simulink model "EPS_sim_test_v1"  (R2019b)
settings: Solver=FixedStepAuto  StartTime=0.0  StopTime=tsimulation  FixedStep=delta_t  MaxStep=10  RelTol=1e-3
values from neighbouring files (symbols this model uses):
  a = 6678    [demoEPS_R2019a.m]    (also in demoEPS_v1.m; demoEPS_v1a.m; demoEPS_v1test.m; demoEPS_v2.m)
  C = Cbat*Nbp*3600    (= 37440)    [demoEPS.m]    (also in demoEPS_R2019a.m; demoEPS_v1.m; demoEPS_v1a.m; demoEPS_v1test.m)
  day = 21    [demoEPS_R2019a.m]    (also in demoEPS_v1.m = 1; demoEPS_v1a.m; demoEPS_v1test.m; demoEPS_v2.m)
  DOD_0 = 0    [demoEPS.m]    (also in demoEPS_R2019a.m; demoEPS_v1.m; demoEPS_v1a.m; demoEPS_v1test.m)
  e = 0.001    [demoEPS_R2019a.m]    (also in demoEPS_v1.m = 0; demoEPS_v1a.m; demoEPS_v1test.m; demoEPS_v2.m)
  hours = 0    [demoEPS_R2019a.m]    (also in demoEPS_v1.m; demoEPS_v1a.m; demoEPS_v1test.m; demoEPS_v2.m)
  i = 51.6    [demoEPS_R2019a.m]    (also in demoEPS_v1.m; demoEPS_v1a.m; demoEPS_v1test.m; demoEPS_v2.m)
  I_BC_max = -input (4)    [battchargedischarge.m]    (also in demoEPS.m = 3; demoEPS_R2019a.m = 3; demoEPS_v1.m = 3; demoEPS_v1a.m = 3)
  I_BD_max = input (3)    [battchargedischarge.m]    (also in demoEPS.m = 5; demoEPS_R2019a.m = 5; demoEPS_v1.m = 5; demoEPS_v1a.m = 5)
  m = 10    [demoEPS_R2019a.m]    (also in demoEPS_v1.m; demoEPS_v1a.m; demoEPS_v1test.m; demoEPS_v2.m)
  minutes = 0    [demoEPS_R2019a.m]    (also in demoEPS_v1.m; demoEPS_v1a.m; demoEPS_v1test.m; demoEPS_v2.m)
  month = 3    [demoEPS_R2019a.m]    (also in demoEPS_v1.m = 1; demoEPS_v1a.m = 6; demoEPS_v1test.m = 12; demoEPS_v2.m)
  Nbs = math.ceil(Vbusmin/Vbatmin)    [calc_mass_EPS.m]    (also in demoEPS.m = 4; demoEPS_R2019a.m = 4; demoEPS_v1.m = 4; demoEPS_v1a.m = 4)
  nu = 0    [demoEPS_R2019a.m]    (also in demoEPS_v1.m; demoEPS_v1a.m; demoEPS_v1test.m; demoEPS_v2.m)
  O = 300    [demoEPS_R2019a.m]    (also in demoEPS_v1.m = 185; demoEPS_v1a.m = 69; demoEPS_v1test.m = 180; demoEPS_v2.m = 243)
  o = 90    [demoEPS_R2019a.m]    (also in demoEPS_v1.m; demoEPS_v1a.m = 150; demoEPS_v1test.m = 150; demoEPS_v2.m)
  P_eps = 0.6    [demoEPS.m]    (also in demoEPS_R2019a.m; demoEPS_v1.m; demoEPS_v1a.m; demoEPS_v1test.m)
  Pload1 = 50    [demoEPS.m]    (also in demoEPS_R2019a.m; demoEPS_v1.m; demoEPS_v1a.m; demoEPS_v1test.m)
  Pload2 = 2    [demoEPS.m]    (also in demoEPS_R2019a.m; demoEPS_v1.m; demoEPS_v1a.m; demoEPS_v1test.m)
  Pload3 = 2.5    [demoEPS.m]    (also in demoEPS_R2019a.m; demoEPS_v1.m; demoEPS_v1a.m; demoEPS_v1test.m)
  Pload4 = 1.7    [demoEPS.m]    (also in demoEPS_R2019a.m; demoEPS_v1.m; demoEPS_v1a.m; demoEPS_v1test.m)
  Psa = 48    [demoEPS.m]    (also in demoEPS_R2019a.m; demoEPS_v1.m; demoEPS_v1a.m; demoEPS_v1test.m)
  seconds = 0    [demoEPS_R2019a.m]    (also in demoEPS_v1.m; demoEPS_v1a.m; demoEPS_v1test.m; demoEPS_v2.m)
  Torbit = 2*pi*sqrt(((h+6378)^3)/398600)/60    [calc_mass_EPS.m]    (also in demoEPS.m = 5400; demoEPS_R2019a.m = 2*pi*sqrt(a^3/(3.986004418E5)); demoEPS_v1.m = 5400; demoEPS_v1a.m = 2*pi*sqrt(a^3/(3.986004418E5)))
  year = 2020    [demoEPS_R2019a.m]    (also in demoEPS_v1.m; demoEPS_v1a.m = 2019; demoEPS_v1test.m = 2019; demoEPS_v2.m)
undefined symbols (not defined in the file or in its folder): km, s
libraries: aerolibconvert2 x6, dspmathops x4, vrlib x3, simulink x2, aerolibutil x2, sharedtransform x1, aerolibgravity2 x1, aerolibcelestial x1
settings Model: Creator=Ricardo  LastModifiedBy=Ricardo

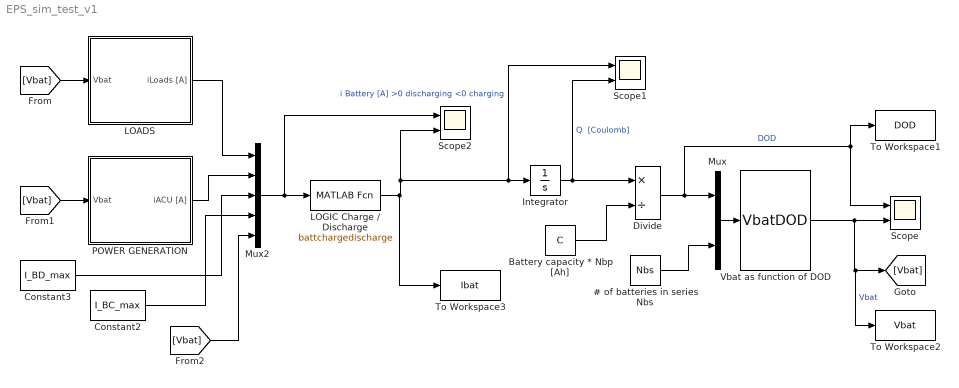
== system EPS_sim_test_v1 ==
  # of batteries in series Nbs : Constant  Value=Nbs
  Battery capacity * Nbp [Ah] : Constant  Value=C
  Constant2 : Constant  Value=I_BC_max
  Constant3 : Constant  Value=I_BD_max
  Divide : Product  Inputs=*/
  Integrator : Integrator  InitialCondition=DOD_0
  LOADS : Subsystem
  LOGIC Charge / Discharge : MATLABFcn  MATLABFcn=battchargedischarge
  Mux : Mux  Inputs=2
  Mux2 : Mux  Inputs=5
  POWER GENERATION : Subsystem
  Scope : Scope  NumInputPorts=2
  Scope1 : Scope  NumInputPorts=2
  Scope2 : Scope  NumInputPorts=2
  To Workspace1 : ToWorkspace  VariableName=DOD  SaveFormat=Timeseries  SampleTime=-1
  To Workspace2 : ToWorkspace  VariableName=Vbat  SaveFormat=Timeseries  SampleTime=-1
  To Workspace3 : ToWorkspace  VariableName=Ibat  SaveFormat=Timeseries  SampleTime=-1
  Vbat as function of DOD : MATLABFcn  MATLABFcn=VbatDOD
  wires:
  Mux/1 -> Vbat as function of DOD/1
  # of batteries in series Nbs/1 -> Mux/2
  Vbat as function of DOD/1 -> To Workspace2/1, [Vbat], Scope/2  "Vbat"
  Divide/1 -> To Workspace1/1, Scope/1, Mux/1  "DOD"
  Integrator/1 -> Scope1/2, Divide/1  "Q  [Coulomb]"
  Battery capacity * Nbp [Ah]/1 -> Divide/2
  [Vbat] -> LOADS/1(Vbat)
  POWER GENERATION/1(iACU [A]) -> Mux2/2
  [Vbat] -> POWER GENERATION/1(Vbat)
  LOADS/1(iLoads [A]) -> Mux2/1
  Mux2/1 -> LOGIC Charge / Discharge/1, Scope2/1
  Constant3/1 -> Mux2/3
  Constant2/1 -> Mux2/4
  LOGIC Charge / Discharge/1 -> To Workspace3/1, Scope1/1, Integrator/1, Scope2/2  "i Battery [A] >0 discharging <0 charging"
  [Vbat] -> Mux2/5

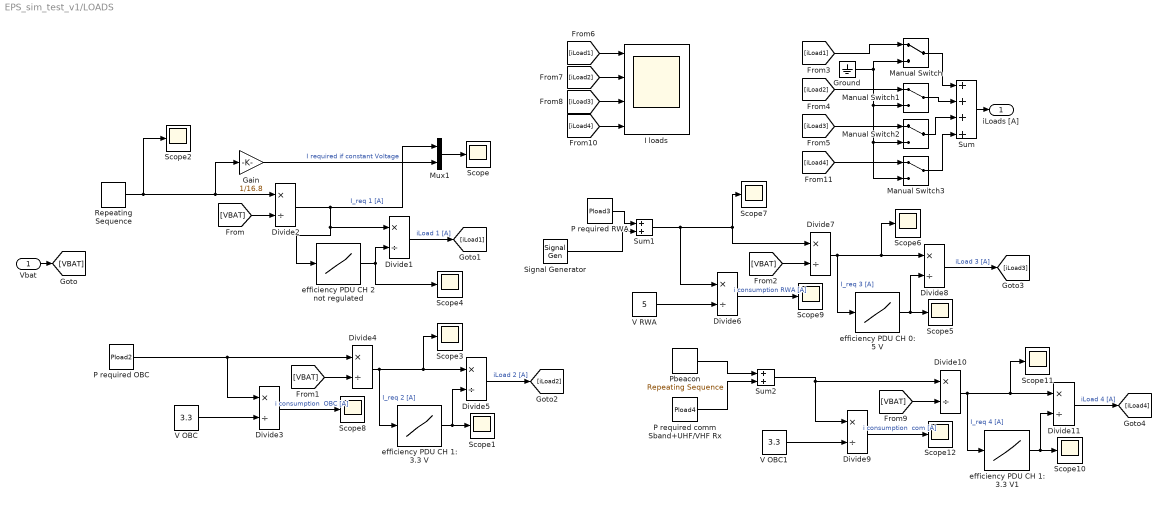
== system EPS_sim_test_v1/LOADS ==
  Vbat : Inport
  Divide{1..11} (11 alike) : Product  Inputs=*/
  Gain : Gain  Gain=1/16.8
  Ground : Ground
  I loads : Scope  NumInputPorts=4
  Manual Switch{,1..3} (4 alike) : ManualSwitch
  Mux1 : Mux  Inputs=2
  P required OBC : Constant  Value=Pload2
  P required RWA : Constant  Value=Pload3
  P required comm Sband+UHF/VHF Rx : Constant  Value=Pload4
  Pbeacon : simulink/Sources/Repeating Sequence  rep_seq_t=[0, 1, 21, 22, 200]  rep_seq_y=[0 3.3 3.3 0 0]
  Repeating Sequence : simulink/Sources/Repeating Sequence  rep_seq_t=[0, 1, (Torbit/2),(Torbit/2)+1, Torbit,2*Torbit,3*Torbit,4*Torbit]  rep_seq_y=[0.32 Pload1 Pload1 0.32 0.32 0.32 0.32 0.32]
  Scope{,1..12} (13 alike) : Scope
  Signal Generator : SignalGenerator  WaveForm=random  Amplitude=0.6  Frequency=0.01
  Sum : Sum  Inputs=++++
  Sum1 : Sum
  Sum2 : Sum
  V OBC : Constant  Value=3.3
  V OBC1 : Constant  Value=3.3
  V RWA : Constant  Value=5
  efficiency PDU CH 0: 5 V : Lookup_n-D  NumberOfTableDimensions=1  BreakpointsForDimension1=[0,0.15,0.18,0.25,0.4,0.5,0.75,1,1.5,2]  Table=[0,0.65,0.7,0.8,0.85,0.88,0.89,0.9,0.88,0.87]  InternalRulePriority=Speed  RndMeth=Simplest  InputSameDT=on
  efficiency PDU CH 1: 3.3 V : Lookup_n-D  NumberOfTableDimensions=1  BreakpointsForDimension1=[0,0.15,0.18,0.25,0.4,0.5,0.75,1,1.5,2]  Table=[0,0.65,0.7,0.8,0.85,0.88,0.89,0.9,0.88,0.87]  InternalRulePriority=Speed  RndMeth=Simplest  InputSameDT=on
  efficiency PDU CH 1: 3.3 V1 : Lookup_n-D  NumberOfTableDimensions=1  BreakpointsForDimension1=[0,0.15,0.18,0.25,0.4,0.5,0.75,1,1.5,2]  Table=[0,0.65,0.7,0.8,0.85,0.88,0.89,0.9,0.88,0.87]  InternalRulePriority=Speed  RndMeth=Simplest  InputSameDT=on
  efficiency PDU CH 2 not regulated : Lookup_n-D  NumberOfTableDimensions=1  BreakpointsForDimension1=[0,0.15,0.2,0.25,0.4,0.5,0.75,1,1.5,2]  Table=[0.25,0.97,0.99,0.98594,0.97572,0.96294,0.95783,0.95783,0.94505,0.93994]  InternalRulePriority=Speed  RndMeth=Simplest  InputSameDT=on
  iLoads [A] : Outport
  wires:
  Gain/1 -> Mux1/2  "I required if constant Voltage"
  Divide2/1 -> Mux1/1, efficiency PDU CH 2 not regulated/1, Divide1/1  "I_req 1 [A]"
  P required OBC/1 -> Divide4/1, Divide3/1
  V OBC/1 -> Divide3/2
  Vbat/1 -> [VBAT]
  [VBAT] -> Divide2/2
  [VBAT] -> Divide4/2
  Divide4/1 -> efficiency PDU CH 1: 3.3 V/1, Scope3/1, Divide5/1  "I_req 2 [A]"
  Sum/1 -> iLoads [A]/1
  Mux1/1 -> Scope/1
  efficiency PDU CH 1: 3.3 V/1 -> Scope1/1, Divide5/2
  Repeating Sequence/1 -> Scope2/1, Gain/1, Divide2/1
  efficiency PDU CH 2 not regulated/1 -> Scope4/1, Divide1/2
  Divide1/1 -> [iLoad1]  "iLoad 1 [A]"
  Divide5/1 -> [iLoad2]  "iLoad 2 [A]"
  V RWA/1 -> Divide6/2
  Divide7/1 -> efficiency PDU CH 0: 5 V/1, Scope6/1, Divide8/1  "I_req 3 [A]"
  efficiency PDU CH 0: 5 V/1 -> Scope5/1, Divide8/2
  [VBAT] -> Divide7/2
  Divide8/1 -> [iLoad3]  "iLoad 3 [A]"
  Manual Switch/1 -> Sum/1
  Manual Switch1/1 -> Sum/2
  Manual Switch2/1 -> Sum/3
  [iLoad2] -> I loads/2
  [iLoad1] -> I loads/1
  [iLoad3] -> I loads/3
  Sum1/1 -> Divide6/1, Divide7/1, Scope7/1
  P required RWA/1 -> Sum1/1
  Signal Generator/1 -> Sum1/2
  Divide3/1 -> Scope8/1  "i consumption  OBC [A]"
  Divide6/1 -> Scope9/1  "i consumption RWA [A]"
  Divide9/1 -> Scope12/1  "i consumption  com [A]"
  [VBAT] -> Divide10/2
  Divide11/1 -> [iLoad4]  "iLoad 4 [A]"
  efficiency PDU CH 1: 3.3 V1/1 -> Scope10/1, Divide11/2
  Divide10/1 -> efficiency PDU CH 1: 3.3 V1/1, Scope11/1, Divide11/1  "I_req 4 [A]"
  Sum2/1 -> Divide9/1, Divide10/1
  V OBC1/1 -> Divide9/2
  [iLoad4] -> I loads/4
  Manual Switch3/1 -> Sum/4
  P required comm Sband+UHF/VHF Rx/1 -> Sum2/2
  Pbeacon/1 -> Sum2/1
  [iLoad4] -> Manual Switch3/1
  [iLoad3] -> Manual Switch2/1
  [iLoad2] -> Manual Switch1/1
  [iLoad1] -> Manual Switch/1
  Ground/1 -> Manual Switch/2, Manual Switch3/2, Manual Switch2/2, Manual Switch1/2

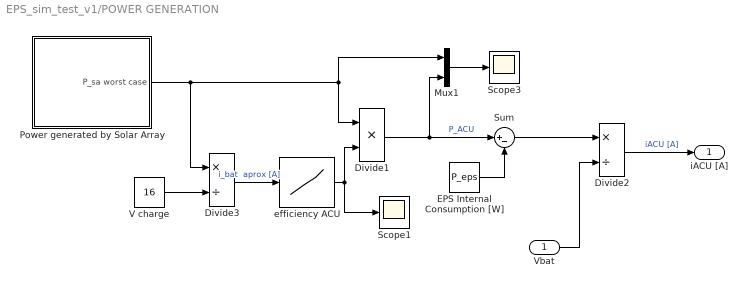
== system EPS_sim_test_v1/POWER GENERATION ==
  Vbat : Inport
  Divide1 : Product  Inputs=**
  Divide2 : Product  Inputs=*/
  Divide3 : Product  Inputs=*/
  EPS Internal Consumption [W] : Constant  Value=P_eps
  Mux1 : Mux  Inputs=2
  Power generated by Solar Array : Subsystem
  Scope1 : Scope
  Scope3 : Scope
  Sum : Sum  Inputs=|+-
  V charge : Constant  Value=16
  efficiency ACU : Lookup_n-D  NumberOfTableDimensions=1  BreakpointsForDimension1=[0,0.15,0.18,0.25,0.4,0.5,0.75,1,1.5,2]  Table=[0,0.59377,0.7,0.75479,0.79162,0.8238,0.85831,0.86406,0.85256,0.84681]  InternalRulePriority=Speed  RndMeth=Simplest  InputSameDT=on
  iACU [A] : Outport
  wires:
  Divide2/1 -> iACU [A]/1  "iACU [A]"
  Mux1/1 -> Scope3/1
  Vbat/1 -> Divide2/2
  efficiency ACU/1 -> Scope1/1, Divide1/2
  Divide1/1 -> Sum/1, Mux1/2  "P_ACU"
  Sum/1 -> Divide2/1
  EPS Internal Consumption [W]/1 -> Sum/2
  Divide3/1 -> efficiency ACU/1  "i_bat  aprox [A]"
  V charge/1 -> Divide3/2
  Power generated by Solar Array/1(P_sa worst case) -> Divide3/1, Mux1/1, Divide1/1

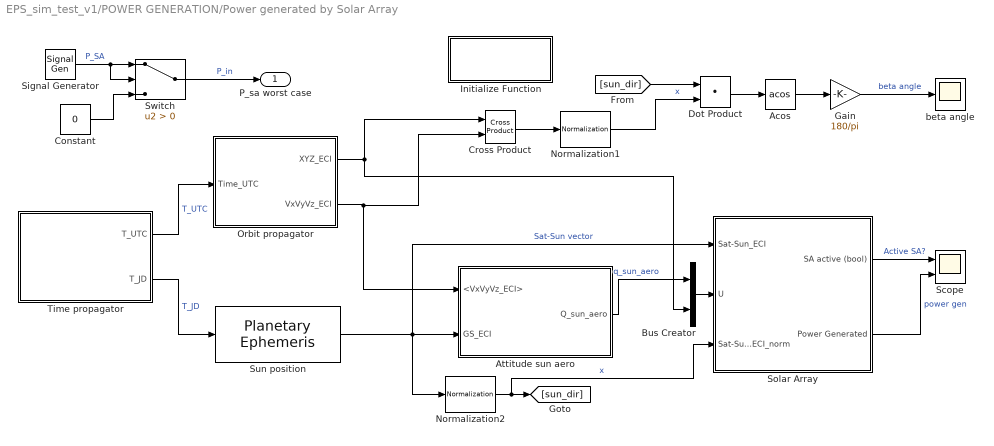
== system EPS_sim_test_v1/POWER GENERATION/Power generated by Solar Array ==
  Acos : Trigonometry  Operator=acos
  Attitude sun aero : Subsystem
  Bus Creator : BusCreator  Inputs=2
  Constant : Constant  Value=0
  Cross Product : vrlib/Utilities/Cross Product
      settings: SourceProductName=Simulink
  Dot Product : DotProduct  InputSameDT=on  OutDataTypeStr=Inherit: Inherit via internal rule
  Gain : Gain  Gain=180/pi
  Initialize Function : Subsystem  TreatAsAtomicUnit=on
  Normalization1 : dspmathops/Normalization  NormType=2-norm  Bias=1e-10  NormOver=Each column  Dimension=1  roundingMode=Floor  overflowMode=off  accumDataTypeStr=Inherit: Same as product output  accumLastDataTypeStr=Inherit: Same as product output  outputDataTypeStr=Inherit: Same as product output  outputMin=[]  outputMax=[]  outputLastDataTypeStr=Inherit: Same as product output
      settings: SourceProductName=DSP System Toolbox
  Normalization2 : dspmathops/Normalization  NormType=2-norm  Bias=1e-10  NormOver=Each column  Dimension=1  roundingMode=Floor  overflowMode=off  accumDataTypeStr=Inherit: Same as product output  accumLastDataTypeStr=Inherit: Same as product output  outputDataTypeStr=Inherit: Same as product output  outputMin=[]  outputMax=[]  outputLastDataTypeStr=Inherit: Same as product output
      settings: SourceProductName=DSP System Toolbox
  Orbit propagator : Subsystem
  Scope : Scope  NumInputPorts=2
  Signal Generator : SignalGenerator  Amplitude=-Psa  Frequency=1/Torbit
  Solar Array : Subsystem
  Sun position : aerolibcelestial/Planetary Ephemeris  kmflag=km,km/s  epochflag=Julian date  de=DE405  nCenter=Earth  nTarget=Sun  errorflag=Error  velflag=off
      settings: SourceProductName=Aerospace Blockset  SourceProductBaseCode=AE
  Switch : Switch  Criteria=u2 > Threshold
  Time propagator : Subsystem
  beta angle : Scope
  P_sa worst case : Outport
  wires:
  Signal Generator/1 -> Switch/2, Switch/1  "P_SA"
  Constant/1 -> Switch/3
  Gain/1 -> beta angle/1  "beta angle"
  Cross Product/1 -> Normalization1/1
  Acos/1 -> Gain/1
  Dot Product/1 -> Acos/1
  Bus Creator/1 -> Solar Array/2(U)
  Orbit propagator/1(XYZ_ECI) -> Cross Product/1, Bus Creator/2
  [sun_dir] -> Dot Product/1
  Time propagator/2(T_JD) -> Sun position/1  "T_JD"
  Normalization2/1 -> Solar Array/3(Sat-Sun_ECI_norm), [sun_dir]  "x"
  Attitude sun aero/1(Q_sun_aero) -> Bus Creator/1  "q_sun_aero"
  Normalization1/1 -> Dot Product/2  "x"
  Time propagator/1(T_UTC) -> Orbit propagator/1("Time_UTC ")  "T_UTC"
  Sun position/1 -> Normalization2/1, Solar Array/1(Sat-Sun_ECI), Attitude sun aero/2(GS_ECI)  "Sat-Sun vector"
  Solar Array/1(SA active (bool)) -> Scope/1  "Active SA?"
  Orbit propagator/2(VxVyVz_ECI) -> Cross Product/2, Attitude sun aero/1(<VxVyVz_ECI>)
  Solar Array/2(Power Generated) -> Scope/2  "power gen"
  Switch/1 -> P_sa worst case/1  "P_in"

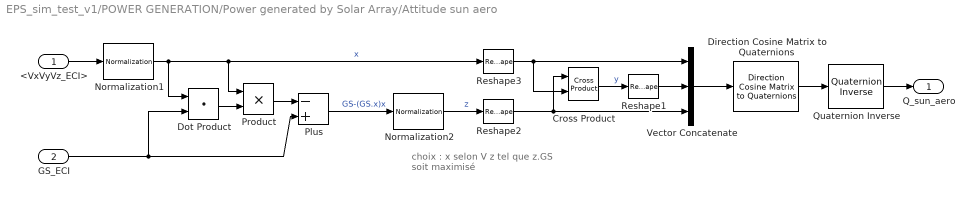
== system EPS_sim_test_v1/POWER GENERATION/Power generated by Solar Array/Attitude sun aero ==
  note: choix :
      | x selon V
      | z tel que z.GS soit maximisé
  <VxVyVz_ECI> : Inport
  GS_ECI : Inport  Port=2
  Cross Product : vrlib/Utilities/Cross Product
      settings: SourceProductName=Simulink
  Direction Cosine Matrix to Quaternions : sharedtransform/Direction Cosine Matrix  to Quaternions  aMode=0  action=None  tolerance=eps(2)
      settings: SourceProductName=Aerospace Blockset  SourceProductBaseCode=AE
  Dot Product : DotProduct  InputSameDT=on  OutDataTypeStr=Inherit: Inherit via internal rule
  Normalization1 : dspmathops/Normalization  NormType=2-norm  Bias=1e-10  NormOver=Each column  Dimension=1  roundingMode=Floor  overflowMode=off  accumDataTypeStr=Inherit: Same as product output  accumLastDataTypeStr=Inherit: Same as product output  outputDataTypeStr=Inherit: Same as product output  outputMin=[]  outputMax=[]  outputLastDataTypeStr=Inherit: Same as product output
      settings: SourceProductName=DSP System Toolbox
  Normalization2 : dspmathops/Normalization  NormType=2-norm  Bias=1e-10  NormOver=Each column  Dimension=1  roundingMode=Floor  overflowMode=off  accumDataTypeStr=Inherit: Same as product output  accumLastDataTypeStr=Inherit: Same as product output  outputDataTypeStr=Inherit: Same as product output  outputMin=[]  outputMax=[]  outputLastDataTypeStr=Inherit: Same as product output
      settings: SourceProductName=DSP System Toolbox
  Plus : Sum  Inputs=-+
  Product : Product
  Quaternion Inverse : aerolibutil/Quaternion Inverse
      settings: SourceProductName=Aerospace Blockset
  Reshape1 : Reshape  OutputDimensionality=Column vector (2-D)
  Reshape2 : Reshape  OutputDimensionality=Column vector (2-D)
  Reshape3 : Reshape  OutputDimensionality=Column vector (2-D)
  Vector Concatenate : Concatenate  NumInputs=3  Mode=Multidimensional array  ConcatenateDimension=2
  Q_sun_aero : Outport  VectorParamsAs1DForOutWhenUnconnected=off
  wires:
  Quaternion Inverse/1 -> Q_sun_aero/1
  Reshape2/1 -> Vector Concatenate/3, Cross Product/1
  Reshape3/1 -> Vector Concatenate/1, Cross Product/2
  Product/1 -> Plus/1
  Dot Product/1 -> Product/2
  Cross Product/1 -> Reshape1/1  "y"
  Normalization2/1 -> Reshape2/1  "z"
  Plus/1 -> Normalization2/1  "GS-(GS.x)x"
  GS_ECI/1 -> Dot Product/2, Plus/2
  Vector Concatenate/1 -> Direction Cosine Matrix to Quaternions/1
  Direction Cosine Matrix to Quaternions/1 -> Quaternion Inverse/1
  Normalization1/1 -> Dot Product/1, Product/1, Reshape3/1  "x"
  <VxVyVz_ECI>/1 -> Normalization1/1
  Reshape1/1 -> Vector Concatenate/2

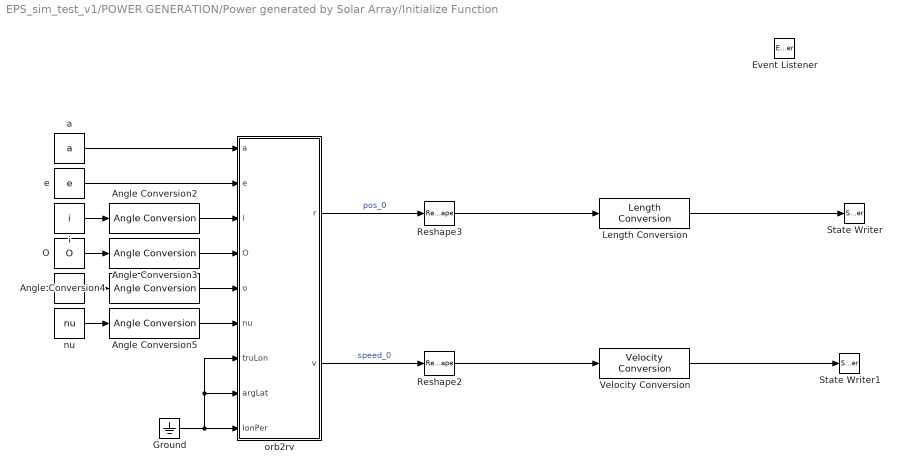
== system EPS_sim_test_v1/POWER GENERATION/Power generated by Solar Array/Initialize Function ==
  Angle Conversion{2..5} (4 alike) : aerolibconvert2/Angle Conversion  IU=deg  OU=rad
  Event Listener : EventListener  DisableCoverage=on  EventName=reset
  Ground : Ground
  Length Conversion : aerolibconvert2/Length Conversion  IU=km  OU=m
  O : Constant  Value=O
  Reshape2 : Reshape  OutputDimensionality=Column vector (2-D)
  Reshape3 : Reshape  OutputDimensionality=Column vector (2-D)
  State Writer : StateWriter  StateOwnerBlock=../../Orbit propagator/Integrator_pos
  State Writer1 : StateWriter  StateOwnerBlock=../../Orbit propagator/Integrator_speed
  Velocity Conversion : aerolibconvert2/Velocity Conversion  IU=km/s  OU=m/s
  a : Constant  Value=a
  e : Constant  Value=e
  i : Constant  Value=i
  nu : Constant  Value=nu
  o : Constant  Value=o
  orb2rv : MATLAB Function  TreatAsAtomicUnit=on
  wires:
  Angle Conversion2/1 -> orb2rv/3(i)
  Length Conversion/1 -> State Writer/1
  Angle Conversion4/1 -> orb2rv/5(o)
  nu/1 -> Angle Conversion5/1
  Angle Conversion3/1 -> orb2rv/4(O)
  e/1 -> orb2rv/2(e)
  Reshape3/1 -> Length Conversion/1
  O/1 -> Angle Conversion3/1
  a/1 -> orb2rv/1(a)
  i/1 -> Angle Conversion2/1
  orb2rv/1(r) -> Reshape3/1  "pos_0"
  o/1 -> Angle Conversion4/1
  Angle Conversion5/1 -> orb2rv/6(nu)
  Velocity Conversion/1 -> State Writer1/1
  Reshape2/1 -> Velocity Conversion/1
  orb2rv/2(v) -> Reshape2/1  "speed_0"
  Ground/1 -> orb2rv/8(argLat), orb2rv/7(truLon), orb2rv/9(lonPer)

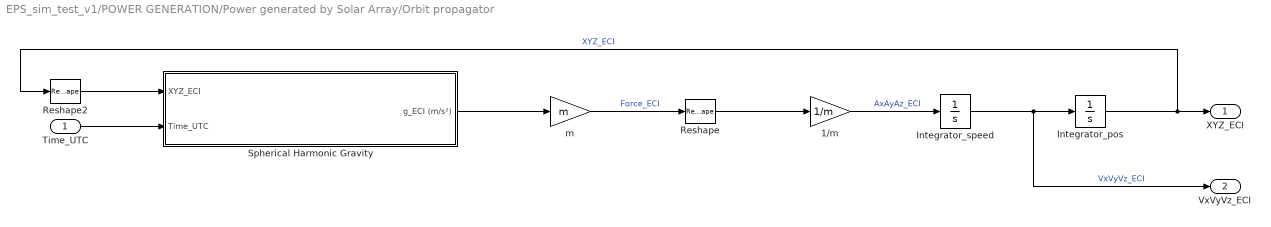
== system EPS_sim_test_v1/POWER GENERATION/Power generated by Solar Array/Orbit propagator ==
  "Time_UTC " : Inport
  1/m : Gain  Gain=1/m
  Integrator_pos : Integrator
  Integrator_speed : Integrator
  Reshape : Reshape  OutputDimensionality=Column vector (2-D)
  Reshape2 : Reshape  OutputDimensionality=Column vector (2-D)
  Spherical Harmonic Gravity : Subsystem  TreatAsAtomicUnit=on  SystemSampleTime=1
  m : Gain  Gain=m
  XYZ_ECI : Outport  VectorParamsAs1DForOutWhenUnconnected=off
  VxVyVz_ECI : Outport  Port=2
  wires:
  Integrator_pos/1 -> Reshape2/1, XYZ_ECI/1  "XYZ_ECI"
  Integrator_speed/1 -> VxVyVz_ECI/1, Integrator_pos/1  "VxVyVz_ECI"
  1/m/1 -> Integrator_speed/1  "AxAyAz_ECI"
  Reshape/1 -> 1/m/1
  m/1 -> Reshape/1  "Force_ECI"
  Spherical Harmonic Gravity/1(g_ECI (m/s²)) -> m/1
  "Time_UTC "/1 -> Spherical Harmonic Gravity/2(Time_UTC)
  Reshape2/1 -> Spherical Harmonic Gravity/1(XYZ_ECI)

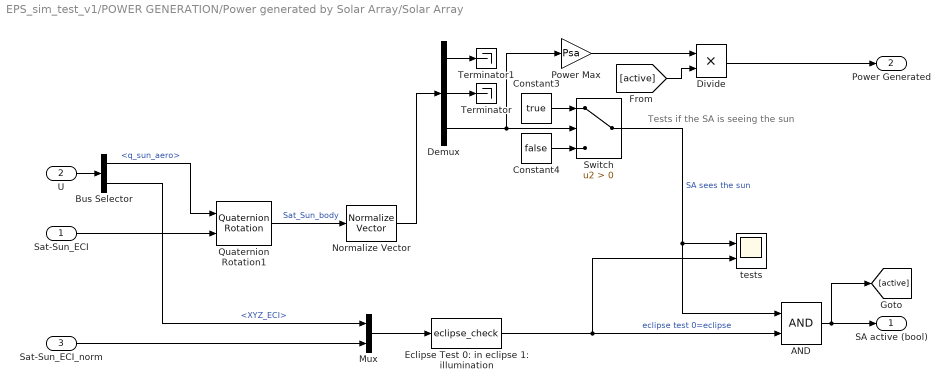
== system EPS_sim_test_v1/POWER GENERATION/Power generated by Solar Array/Solar Array ==
  note: Tests if the SA is seeing the sun
  Sat-Sun_ECI : Inport
  U : Inport  Port=2
  Sat-Sun_ECI_norm : Inport  Port=3
  AND : Logic  IconShape=distinctive  AllPortsSameDT=off  OutDataTypeStr=boolean
  Bus Selector : BusSelector  OutputSignals=q_sun_aero,XYZ_ECI
  Constant3 : Constant  Value=true
  Constant4 : Constant  Value=false
  Demux : Demux  Outputs=3
  Divide : Product  Inputs=**
  Eclipse Test 0: in eclipse 1: illumination : MATLABFcn  MATLABFcn=eclipse_check
  Mux : Mux  Inputs=2
  Normalize Vector : vrlib/Utilities/Normalize Vector  maxzero=0
      settings: SourceProductName=Simulink
  Power Max : Gain  Gain=Psa
  Quaternion Rotation1 : aerolibutil/Quaternion Rotation
  Switch : Switch  Criteria=u2 > Threshold
  Terminator : Terminator
  Terminator1 : Terminator
  tests : Scope  NumInputPorts=2
  SA active (bool) : Outport  VectorParamsAs1DForOutWhenUnconnected=off
  Power Generated : Outport  Port=2
  wires:
  Switch/1 -> AND/1, tests/1  "SA sees the sun"
  U/1 -> Bus Selector/1
  Sat-Sun_ECI/1 -> Quaternion Rotation1/2
  Bus Selector/1 -> Quaternion Rotation1/1  "<q_sun_aero>"
  Quaternion Rotation1/1 -> Normalize Vector/1  "Sat_Sun_body"
  Demux/3 -> Power Max/1, Switch/2
  Constant3/1 -> Switch/1
  Demux/2 -> Terminator/1
  Demux/1 -> Terminator1/1
  Bus Selector/2 -> Mux/1  "<XYZ_ECI>"
  AND/1 -> SA active (bool)/1, [active]
  Constant4/1 -> Switch/3
  Normalize Vector/1 -> Demux/1
  Divide/1 -> Power Generated/1
  Power Max/1 -> Divide/1
  [active] -> Divide/2
  Sat-Sun_ECI_norm/1 -> Mux/2
  Mux/1 -> Eclipse Test 0: in eclipse 1: illumination/1
  Eclipse Test 0: in eclipse 1: illumination/1 -> AND/2, tests/2  "eclipse test 0=eclipse"

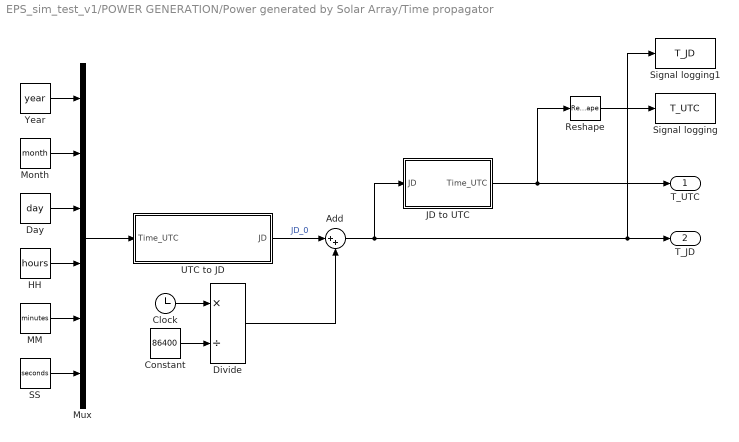
== system EPS_sim_test_v1/POWER GENERATION/Power generated by Solar Array/Time propagator ==
  Add : Sum  Inputs=|++
  Clock : Clock
  Constant : Constant  Value=86400
  Day : Constant  Value=day
  Divide : Product  Inputs=*/
  HH : Constant  Value=hours
  JD to UTC : MATLAB Function  TreatAsAtomicUnit=on
  MM : Constant  Value=minutes
  Month : Constant  Value=month
  Mux : Mux  Inputs=6
  Reshape : Reshape
  SS : Constant  Value=seconds
  Signal logging : ToWorkspace  VariableName=T_UTC  SaveFormat=Timeseries  SampleTime=1
      settings: Save2DSignal=2-D array (concatenate along first dimension)
  Signal logging1 : ToWorkspace  VariableName=T_JD  SaveFormat=Timeseries  SampleTime=1
      settings: Save2DSignal=2-D array (concatenate along first dimension)
  UTC to JD : MATLAB Function  TreatAsAtomicUnit=on
  Year : Constant  Value=year
  T_UTC : Outport  VectorParamsAs1DForOutWhenUnconnected=off
  T_JD : Outport  Port=2  VectorParamsAs1DForOutWhenUnconnected=off
  wires:
  UTC to JD/1(JD) -> Add/1  "JD_0"
  Clock/1 -> Divide/1
  Constant/1 -> Divide/2
  JD to UTC/1(Time_UTC) -> T_UTC/1, Reshape/1
  Divide/1 -> Add/2
  Mux/1 -> UTC to JD/1(Time_UTC)
  Day/1 -> Mux/3
  Month/1 -> Mux/2
  Year/1 -> Mux/1
  HH/1 -> Mux/4
  MM/1 -> Mux/5
  SS/1 -> Mux/6
  Reshape/1 -> Signal logging/1
  Add/1 -> Signal logging1/1, T_JD/1, JD to UTC/1(JD)

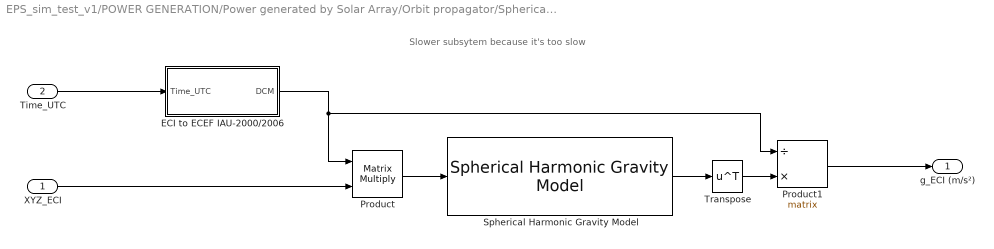
== system EPS_sim_test_v1/POWER GENERATION/Power generated by Solar Array/Orbit propagator/Spherical Harmonic Gravity ==
  note: Slower subsytem because it's too slow
  XYZ_ECI : Inport
  Time_UTC : Inport  Port=2
  ECI to ECEF IAU-2000/2006 : MATLAB Function  TreatAsAtomicUnit=on
  Product : Product  Multiplication=Matrix(*)
  Product1 : Product  Inputs=/*  Multiplication=Matrix(*)
  Spherical Harmonic Gravity Model : aerolibgravity2/Spherical Harmonic Gravity Model  units=Metric (MKS)  degree=100  action=Warning  ptype=EGM2008  datafile='aerogmm2b.mat'
      settings: SourceProductName=Aerospace Blockset  SourceProductBaseCode=AE
  Transpose : Math  Operator=transpose  SaturateOnIntegerOverflow=on
  g_ECI (m/s²) : Outport
  wires:
  ECI to ECEF IAU-2000/2006/1(DCM) -> Product1/1, Product/1
  Transpose/1 -> Product1/2
  Product/1 -> Spherical Harmonic Gravity Model/1
  Spherical Harmonic Gravity Model/1 -> Transpose/1
  XYZ_ECI/1 -> Product/2
  Product1/1 -> g_ECI (m/s²)/1
  Time_UTC/1 -> ECI to ECEF IAU-2000/2006/1(Time_UTC)

== matlab function EPS_sim_test_v1/POWER GENERATION/Power generated by Solar Array/Time propagator/JD to UTC ==
  data: JD input; Time_UTC output
function Time_UTC = fcn(JD)
    coder.extrinsic('datetime','datevec');
    Time_UTC = [0,0,0,0,0,0];
Time_UTC =  datevec(datetime(JD,'convertfrom','juliandate'));

== matlab function EPS_sim_test_v1/POWER GENERATION/Power generated by Solar Array/Time propagator/UTC to JD ==
  data: Time_UTC input; JD output
function JD = fcn(Time_UTC)

% JD = juliandate(Time_UTC);
JD = Dt2jD(Time_UTC);

== matlab function EPS_sim_test_v1/POWER GENERATION/Power generated by Solar Array/Initialize Function/orb2rv ==
  data: a input; r output; e input; i input; O input; o input; nu input; v output; truLon input; argLat input; lonPer input
%----------------------- Begin Code Sequence -----------------------------%
% Purpose:                                                                %
% Convert a given set of Keplerian Orbital Elements to state vectors in   %
% in the ECI frame of reference                                           %
%                                                                         %
%-------------------------------------------------------------------------%
%                                                                         %
% Inputs:                                                                 %
%-------- 
%a                      [1 x N]                         Semimajor axis
%                                                       (km)
%
%e                      [1 x N]                         Eccentricity Magnitude
%                                                       (unitless)
%
%i                      [1 x N]                         inclination
%                                                       (radians)
%
%O                      [1 x N]                         Right Ascention of
%                                                       the ascending node
%                                                       (radians)
%
%o                      [1 x N]                         Argument of perigee
%                                                       (radians)
%
%nu                     [1 x N]                         True Anomaly
%                                                       (radians)
%
%truLon                 [1 x N]                         True Longitude
%                                                       (radians)
%
%argLat                 [1 x N]                         Argument of Latitude
%                                                       (radians)
%
%lonPer                 [1 x N]                         Longitude of Periapse
%                                                       (radians)
%
%mu                     double                          Gravitational Constant
%                                                       Defaults to Earth if
%                                                       not specified
%
% Outputs:
%---------                                                                %
%r_ECI                  [3 x N]                         Position Vector in
%                                                       ECI coordinate
%                                                       frame of reference
%
%v_ECI                  [3 x N]                         Velocity vector in
%                                                       ECI coordinate
%                                                       frame of reference
%
% References:
%-------------
%Vallado,D. Fundamentals of Astrodynamics and Applications. 2007.
%
% Function Dependencies:
%------------------
%None
%------------------------------------------------------------------       %
% Programed by Darin Koblick  03-04-2012                                  %
%------------------------------------------------------------------       %
function [r,v] = orb2rv(a,e,i,O,o,nu,truLon,argLat,lonPer)
mu = 398600.4418;
%Make all inputs consistent w/ dimensions
a = a(:); e = e(:); i = i(:); O = O(:); o = o(:); nu = nu(:);
if e<1
    p=a*(1-e*e);
else
    p=2*a;
end
ietol = 1e-8;
idx = e < ietol & mod(i,pi) < ietol;
if any(idx); o(idx) = 0; O(idx) = 0; nu(idx) = truLon(idx); end
idx = e < ietol & mod(i,pi) > ietol;
if any(idx); o(idx) = 0; nu(idx) = argLat(idx); end
idx = e > ietol & mod(i,pi) < ietol;
if any(idx); O(idx) = 0; o(idx) = lonPer(idx); end
%Find rPQW and vPQW
rPQW = cat(2,p.*cos(nu)./(1 +e.*cos(nu)),p.*sin(nu)./(1+e.*cos(nu)),zeros(size(nu)));
vPQW = cat(2,-sqrt(mu./p).*sin(nu),sqrt(mu./p).*(e+cos(nu)),zeros(size(nu)));
%Create Transformation Matrix
PQW2IJK = NaN(3,3,size(p,1));
cO = cos(O); sO = sin(O); co = cos(o); so = sin(o); ci = cos(i); si = sin(i);
PQW2IJK(1,1,:) = cO.*co-sO.*so.*ci; PQW2IJK(1,2,:) = -cO.*so-sO.*co.*ci; PQW2IJK(1,3,:) = sO.*si;
PQW2IJK(2,1,:) = sO.*co+cO.*so.*ci; PQW2IJK(2,2,:) = -sO.*so+cO.*co.*ci; PQW2IJK(2,3,:) = -cO.*si;
PQW2IJK(3,1,:) = so.*si;            PQW2IJK(3,2,:) = co.*si;             PQW2IJK(3,3,:) = ci;
%Transform rPQW and vPQW to rECI and vECI
r = multiDimMatrixMultiply(PQW2IJK,rPQW)';  
v = multiDimMatrixMultiply(PQW2IJK,vPQW)';
end
function c = multiDimMatrixMultiply(a,b)
c = NaN(size(b));
c(:,1) = sum(bsxfun(@times,a(1,:,:),permute(b,[3 2 1])),2);
c(:,2) = sum(bsxfun(@times,a(2,:,:),permute(b,[3 2 1])),2);
c(:,3) = sum(bsxfun(@times,a(3,:,:),permute(b,[3 2 1])),2);
end

== matlab function EPS_sim_test_v1/POWER GENERATION/Power generated by Solar Array/Orbit propagator/Spherical Harmonic Gravity/ECI to ECEF IAU-2000//2006 ==
  data: Time_UTC input; DCM output
function DCM = fcn(Time_UTC)
    coder.extrinsic('dcmeci2ecef');
    DCM = zeros(3,3);
DCM = dcmeci2ecef('IAU-2000/2006',Time_UTC);
